simulink library "avlAerodynamics2D_ul"  (R2018b)
settings: Solver=VariableStepAuto  StartTime=0.0  StopTime=10.0  RelTol=1e-3
undefined symbols (not defined in the file or in its folder): CDTable, CLTable, CMxTable, CMyTable, CMzTable, CS_gain
settings Model: Creator=mcobb  LastModifiedBy=mcobb

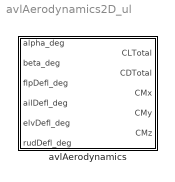
== system avlAerodynamics2D_ul ==
  avlAerodynamics : Subsystem  mask{CLTable=CLTable, CDTable=CDTable, CMxTable=CMxTable, CMyTable=CMyTable, CMzTable=CMzTable, CS_gain=CS_gain}
      mask prompts: CLTable "CL lookup table object"; CDTable "CD lookup table object"; CMxTable "CMx lookup table object"; CMyTable "CMy lookup table object"; CMzTable "CMz lookup table object"; CS_gain "Control surface gain matrix"

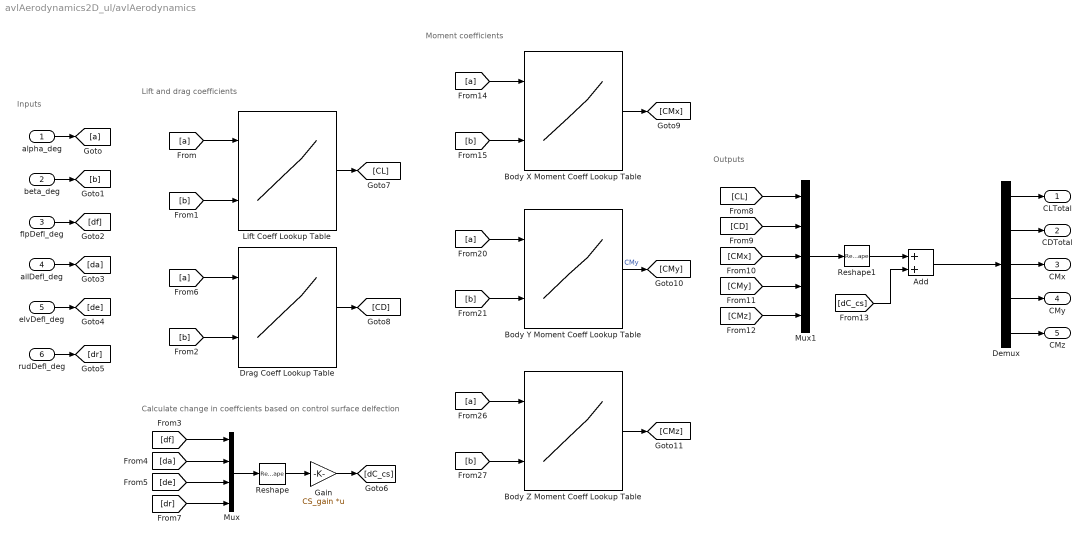
== system avlAerodynamics2D_ul/avlAerodynamics ==
  note: Outputs
  note: Calculate change in coeffcients based on control surface
      | delfection
  note: Inputs
  note: Lift and drag coefficients
  note: Moment coefficients
  alpha_deg : Inport
  beta_deg : Inport  Port=2
  flpDefl_deg : Inport  Port=3
  ailDefl_deg : Inport  Port=4
  elvDefl_deg : Inport  Port=5
  rudDefl_deg : Inport  Port=6
  Add : Sum
  Body X Moment Coeff Lookup Table : Lookup_n-D  DataSpecification=Lookup table object  LookupTableObject=CMxTable  BreakpointsForDimension3=[5, 7]  Table=reshape(repmat([4 5 6;16 19 20;10 18 23],1,2),[3,3,2])  InternalRulePriority=Speed  RndMeth=Simplest  InputSameDT=on
  Body Y Moment Coeff Lookup Table : Lookup_n-D  DataSpecification=Lookup table object  LookupTableObject=CMyTable  BreakpointsForDimension3=[5, 7]  Table=reshape(repmat([4 5 6;16 19 20;10 18 23],1,2),[3,3,2])  InternalRulePriority=Speed  RndMeth=Simplest  InputSameDT=on
  Body Z Moment Coeff Lookup Table : Lookup_n-D  DataSpecification=Lookup table object  LookupTableObject=CMzTable  BreakpointsForDimension3=[5, 7]  Table=reshape(repmat([4 5 6;16 19 20;10 18 23],1,2),[3,3,2])  InternalRulePriority=Speed  RndMeth=Simplest  InputSameDT=on
  Demux : Demux  Outputs=5
  Drag Coeff Lookup Table : Lookup_n-D  DataSpecification=Lookup table object  LookupTableObject=CDTable  BreakpointsForDimension3=[5, 7]  Table=reshape(repmat([4 5 6;16 19 20;10 18 23],1,2),[3,3,2])  InternalRulePriority=Speed  RndMeth=Simplest  InputSameDT=on
  Gain : Gain  Gain=CS_gain  Multiplication=Matrix(K*u)
  Lift Coeff Lookup Table : Lookup_n-D  DataSpecification=Lookup table object  LookupTableObject=CLTable  BreakpointsForDimension3=[5, 7]  Table=reshape(repmat([4 5 6;16 19 20;10 18 23],1,2),[3,3,2])  InternalRulePriority=Speed  RndMeth=Simplest  InputSameDT=on
  Mux : Mux
  Mux1 : Mux  Inputs=5
  Reshape : Reshape  OutputDimensionality=Column vector (2-D)
  Reshape1 : Reshape  OutputDimensionality=Column vector (2-D)
  CLTotal : Outport
  CDTotal : Outport  Port=2
  CMx : Outport  Port=3
  CMy : Outport  Port=4
  CMz : Outport  Port=5
  wires:
  alpha_deg/1 -> [a]
  beta_deg/1 -> [b]
  flpDefl_deg/1 -> [df]
  ailDefl_deg/1 -> [da]
  elvDefl_deg/1 -> [de]
  rudDefl_deg/1 -> [dr]
  [b] -> Lift Coeff Lookup Table/2
  [a] -> Lift Coeff Lookup Table/1
  [a] -> Drag Coeff Lookup Table/1
  [b] -> Drag Coeff Lookup Table/2
  Reshape/1 -> Gain/1
  [dr] -> Mux/4
  [de] -> Mux/3
  [da] -> Mux/2
  [df] -> Mux/1
  Mux/1 -> Reshape/1
  Gain/1 -> [dC_cs]
  [a] -> Body X Moment Coeff Lookup Table/1
  [b] -> Body Z Moment Coeff Lookup Table/2
  [b] -> Body X Moment Coeff Lookup Table/2
  [a] -> Body Z Moment Coeff Lookup Table/1
  [b] -> Body Y Moment Coeff Lookup Table/2
  [a] -> Body Y Moment Coeff Lookup Table/1
  Lift Coeff Lookup Table/1 -> [CL]
  Drag Coeff Lookup Table/1 -> [CD]
  Body X Moment Coeff Lookup Table/1 -> [CMx]
  Body Y Moment Coeff Lookup Table/1 -> [CMy]  "CMy"
  Body Z Moment Coeff Lookup Table/1 -> [CMz]
  [CMx] -> Mux1/3
  [CL] -> Mux1/1
  [CD] -> Mux1/2
  [CMy] -> Mux1/4
  [CMz] -> Mux1/5
  Mux1/1 -> Reshape1/1
  Reshape1/1 -> Add/1
  [dC_cs] -> Add/2
  Add/1 -> Demux/1
  Demux/2 -> CDTotal/1
  Demux/1 -> CLTotal/1
  Demux/3 -> CMx/1
  Demux/4 -> CMy/1
  Demux/5 -> CMz/1
